simulink model "sl_drivepoint"  (R2022a)
settings: Solver=ode45  StartTime=0.0  StopTime=10.0  RelTol=1e-3  EnableMultiTasking=on
InitFcn:
  | if exist('x0')
  |   assert(length(x0)==3, 'x0 must be a 3 vector');
  | else
  |   x0 = [5 5 0];
  |   msgbox(sprintf('x0 not defined in workspace, setting it to [%g %g %g]\n', x0));
  | end
  | if exist('xg')
  |   assert(length(xg)==2, 'xg must be a 2 vector');
  | else
  |   xg = [0 0];
  |   msgbox(sprintf('xg not defined in workspace, setting it to [%g %g]\n', xg));
  | end
  | % clean up old vehicle icons
  | set(0, 'ShowHiddenHandles', 'on')
  | delete(findobj('Tag', 'vehicle'))
  | set(0, 'ShowHiddenHandles', 'off')
  | clear out
StopFcn:
  | % update the XY scope
  | if exist('out')
  |  % come here if running interactively, the output variable has been
  |  % saved to the workspace
  |   set(0, 'ShowHiddenHandles', 'on')
  |   fig = findobj('name', 'XY');
  |   ax = findobj(fig, 'type', 'axes');
  |   axes(ax);
  |   grid on
  |   hold on
  |   plot_vehicle(x0, 'r', 'Tag', 'vehicle')
  |   plot_vehicle(out.y(end,:), 'b', 'Tag', 'vehicle')
  |   hold off
  |   set(0, 'ShowHiddenHandles', 'off')
  | end
libraries: robotmobilelib x1, roblocks x1, simulink x1
settings Model: Creator=pic  LastModifiedBy=rpill
settings SolverCC: AlgebraicLoopSolver=TrustRegion  MaxZcPerStep=1
settings DataIOCC: SaveFormat=Array  TimeSaveName=t  OutputSaveName=y
settings OptimizationCC: ExpressionDepthLimit=2147483647  LifeSpan=inf
settings DebuggingCC: UnderspecifiedInitializationDetection=Classic  MergeDetectMultiDrivingBlocksExec=none  UnconnectedInputMsg=warning  UnconnectedOutputMsg=warning  UnconnectedLineMsg=warning  AllowSymbolicDim=off  StateNameClashWarn=warning  SFUnexpectedBacktrackingDiag=warning  SFNoUnconditionalDefaultTransitionDiag=warning  SFExecutionAtInitializationDiag=none  SFMachineParentedDataDiag=warning  ArithmeticOperatorsInVariantConditions=warning
settings HardwareCC: ProdBitPerPointer=32  ProdBitPerSizeT=32  ProdBitPerPtrDiffT=32  ProdLargestAtomicFloat=None  ProdIntDivRoundTo=Undefined  ProdEndianess=Unspecified  ProdWordSize=32  ProdHWDeviceType=32-bit Generic
settings ModelReferenceCC: PropagateSignalLabelsOutOfModel=off
settings SFSimCC: SimUseLocalCustomCode=off  CustomCodeUndefinedFunction=UseInterfaceOnly
settings RTWCC: RTWUseLocalCustomCode=off  DLArmComputeVersion=19.05
settings CodeAppCC: StateflowObjectComments=on
settings GRTTargetCC: TargetLangStandard=C89/C90 (ANSI)  CombineOutputUpdateFcns=off  GRTInterface=on
settings ConfigComp: CovMetricSettings=dw  CovSaveCumulativeToWorkspaceVar=on  CovSaveSingleToWorkspaceVar=on  CovExternalEMLEnable=off

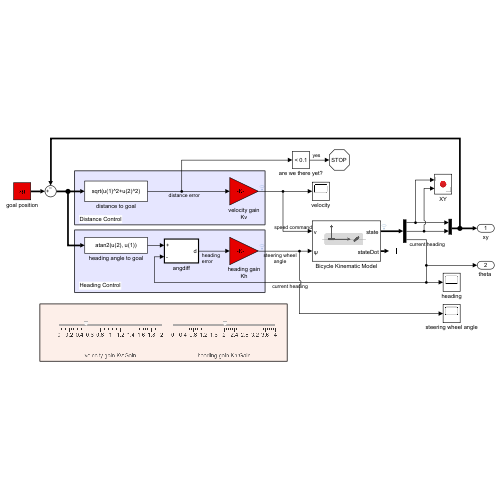
[thumbnail: Simulink's stored preview of the top-level diagram]
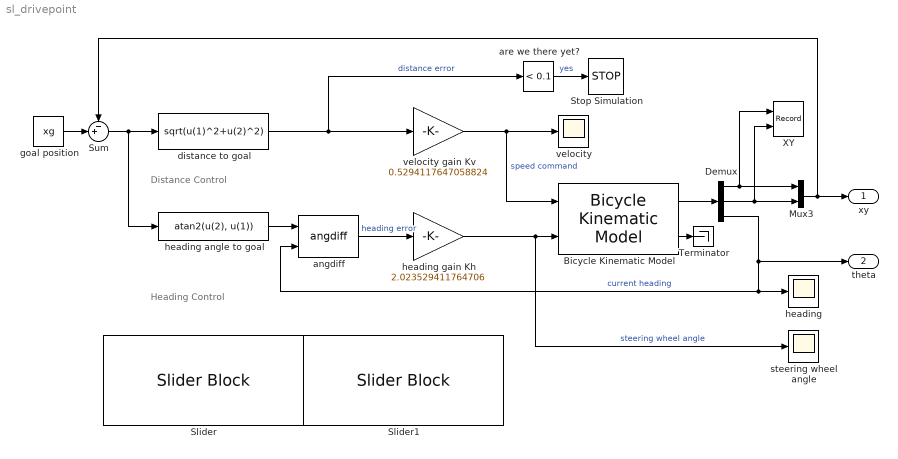
== system sl_drivepoint ==
  note: Distance Control
  note: Heading Control
  Bicycle Kinematic Model : robotmobilelib/Bicycle Kinematic Model  VehicleInputs=Vehicle Speed & Steering Angle  WheelBase=1  VehicleSpeedRange=[0 1]  MaxSteeringAngle=1  InitialState=x0  SimulateUsing=Interpreted execution
      settings: SourceProductBaseCode=RO
  Demux : Demux  Outputs=3
  Mux3 : Mux  Inputs=2
  Slider : SliderBlock  LabelPosition=Bottom  ScaleMax=2
  Slider1 : SliderBlock  LabelPosition=Bottom  ScaleMax=4
  Stop Simulation : Stop
  Sum : Sum  Inputs=-+|
  Terminator : Terminator
  XY : Record  FileSettingsInternal="{\"entries\":[{\"content\":{\"excelSettings\":{\"content\":{},\"type\":\"Streamout.ExcelSettings\"}},\"type\":\"Streamout.FileSettingStorage\",\"uuid\":\"c94ec0ea-23e6-47f1-afe2-3dc06345a3b1\"}],\"packageUris\":[\"http://schema.mathworks.com/mf0/streamout_blocks/R2020a\"],\"version\":\"1.0\"}"  Layout=[1 1]  SignalsInternal="{\"entries\":[{\"content\":{\"signals\":[{\"content\":{\"blockPath\":[\"sl_drivepoint/XY\"],\"channel\":[],\"dimensions\":[1],\"domain\":\"sl_drivepoint/XY\",\"lineColor\":\"#a2142f\",\"plots\":[1],\"port\":1,\"sid\":[],\"signalID\":118,\"signalName\":\"XY Graph:1\"},\"type\":\"RecordBlkView.Signal\",\"uuid\":\"a536fea5-b545-404d-9c96-703ac1270b99\"},{\"content\":{\"blockPath\":[\"sl_drivepoint/XY\"],\"channel\":[],\"dimensions\":[1],\"domain\":\"sl_drivepoint/XY\",\"lineColor\":\"#139fff\",\"plots\":[1],\"port\":2,\"sid\":[],\"signalID\":121,\"signalName\":\"XY Graph:2\"},\"type\":\"RecordBlkView.Signal\",\"uuid\":\"794a2895-7772-4362-91e3-837c6f1cdbb3\"}]},\"type\":\"RecordBlkView.InputSignals\",\"uuid\":\"6ebc5a27-5272-42a2-92a1-fc863dbda38b\"}],\"packageUris\":[\"http://schema.mathworks.com/mf0/streamout_blocks/R2020a\"],\"version\":\"1.0\"}"  VisualizationBindings="{\"xyplotplugin\":{\"info\":[{\"series\":[{\"bindingParametersList\":[{\"parameter\":\"X-Axis\",\"signalID\":118,\"signalName\":\"XY Graph:1\"},{\"parameter\":\"Y-Axis\",\"signalID\":121,\"signalName\":\"XY Graph:2\"}],\"seriesID\":9203}],\"subplotID\":1}]}}"  CompatibilityTag=XY  st=-1
  angdiff : roblocks/angdiff  SystemSampleTime=-1  VariantActivationTime=update diagram  Latency=0  AutoFrameSizeCalculation=off
  are we there yet? : simulink/Logic and Bit Operations/Compare To Constant  relop=<  const=0.1  OutDataTypeStr=boolean
  distance to goal : Fcn  Expr=sqrt(u(1)^2+u(2)^2)
  goal position : Constant  Value=xg
  heading : Scope
  heading angle to goal : Fcn  Expr=atan2(u(2), u(1))
  heading gain Kh : Gain  Gain=2.023529411764706
  steering wheel angle : Scope
  velocity : Scope
  velocity gain Kv : Gain  Gain=0.5294117647058824
  xy : Outport  VectorParamsAs1DForOutWhenUnconnected=off
  "theta " : Outport  Port=2  VectorParamsAs1DForOutWhenUnconnected=off
  wires:
  Demux/1 -> XY/1, Mux3/1
  Demux/2 -> XY/2, Mux3/2
  Mux3/1 -> xy/1, Sum/1
  Sum/1 -> distance to goal/1, heading angle to goal/1
  distance to goal/1 -> velocity gain Kv/1, are we there yet?/1  "distance error"
  heading angle to goal/1 -> angdiff/1
  Demux/3 -> angdiff/2, heading/1, "theta "/1  "current heading"
  velocity gain Kv/1 -> Bicycle Kinematic Model/1, velocity/1  "speed command"
  goal position/1 -> Sum/2
  heading gain Kh/1 -> steering wheel angle/1, Bicycle Kinematic Model/2  "steering wheel angle"
  are we there yet?/1 -> Stop Simulation/1  "yes"
  Bicycle Kinematic Model/1 -> Demux/1
  Bicycle Kinematic Model/2 -> Terminator/1
  angdiff/1 -> heading gain Kh/1  "heading error"
